simulink model "manual_model_ol"  (R2018a)
settings: Solver=VariableStepAuto  StartTime=0.0  StopTime=30.0  RelTol=1e-3
undefined symbols (not defined in the file): A_real, B_real, C_real
settings Model: Creator=Blake  LastModifiedBy=Blake

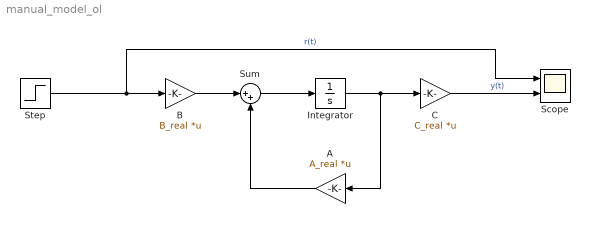
== system manual_model_ol ==
  A : Gain  Gain=A_real  Multiplication=Matrix(K*u)
  B : Gain  Gain=B_real  Multiplication=Matrix(K*u)
  C : Gain  Gain=C_real  Multiplication=Matrix(K*u)
  Integrator : Integrator
  Scope : Scope  NumInputPorts=2
  Step : Step  After=70  SampleTime=0
  Sum : Sum  Inputs=|++
  wires:
  Sum/1 -> Integrator/1
  Step/1 -> Scope/1, B/1  "r(t)"
  C/1 -> Scope/2  "y(t)"
  B/1 -> Sum/1
  Integrator/1 -> A/1, C/1
  A/1 -> Sum/2
